simulink model "DeltaQuad"  (Simulink 9.1)
settings: Solver=VariableStepAuto  StartTime=0.0  StopTime=10.0  RelTol=1e-3
settings Model: Creator=PSere  LastModifiedBy=PSere
settings DataIOCC: SaveFormat=Dataset
settings OptimizationCC: LifeSpan=auto
settings DebuggingCC: UnderspecifiedInitializationDetection=Simplified  MergeDetectMultiDrivingBlocksExec=error  SFUnexpectedBacktrackingDiag=error  SFNoUnconditionalDefaultTransitionDiag=error  SFExecutionAtInitializationDiag=warning
settings HardwareCC: ProdBitPerPointer=64  ProdBitPerSizeT=64  ProdBitPerPtrDiffT=64  ProdLargestAtomicFloat=Float  ProdIntDivRoundTo=Zero  ProdEndianess=LittleEndian  ProdWordSize=64  ProdHWDeviceType=Intel->x86-64 (Windows64)
settings ModelReferenceCC: PropagateSignalLabelsOutOfModel=on
settings CodeAppCC: StateflowObjectComments=off
settings GRTTargetCC: TargetLangStandard=C99 (ISO)  CombineOutputUpdateFcns=on  GRTInterface=off
settings ConfigComp: CovMetricSettings=dwe  CovHtmlReporting=off  CovSaveCumulativeToWorkspaceVar=off  CovSaveSingleToWorkspaceVar=off  CovExternalEMLEnable=on

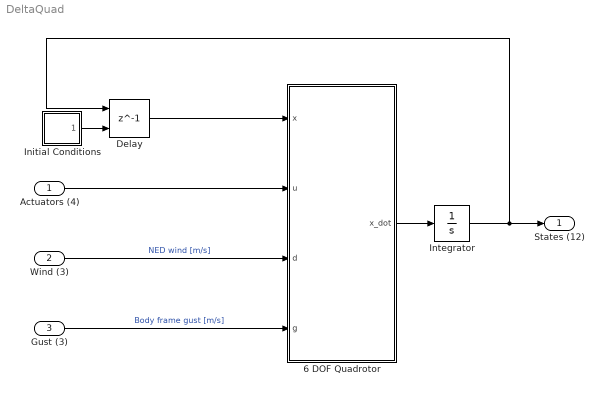
== system DeltaQuad ==
  Actuators (4) : Inport
  Wind (3) : Inport  Port=2
  Gust (3) : Inport  Port=3
  6 DOF Quadrotor : MATLAB Function  TreatAsAtomicUnit=on
  Delay : Delay  DelayLength=1  InitialConditionSource=Input port
      settings: InputPortMap=u0,p4
  "Initial Conditions " : Subsystem  mask{Pn=0, Pe=0, Pd=0, u=0, v=0, w=0, phi=0, theta=0, psi=0, p=0, q=0, r=0}
      mask prompts: Pn "Position North"; Pe "Position East"; Pd "Position Down"
  Integrator : Integrator
  States (12) : Outport
  wires:
  Actuators (4)/1 -> 6 DOF Quadrotor/2(u)
  Wind (3)/1 -> 6 DOF Quadrotor/3(d)  "NED wind [m/s]"
  Delay/1 -> 6 DOF Quadrotor/1(x)
  6 DOF Quadrotor/1(x_dot) -> Integrator/1
  Integrator/1 -> Delay/1, States (12)/1
  "Initial Conditions "/1(IC (12)) -> Delay/2
  Gust (3)/1 -> 6 DOF Quadrotor/4(g)  "Body frame gust [m/s]"

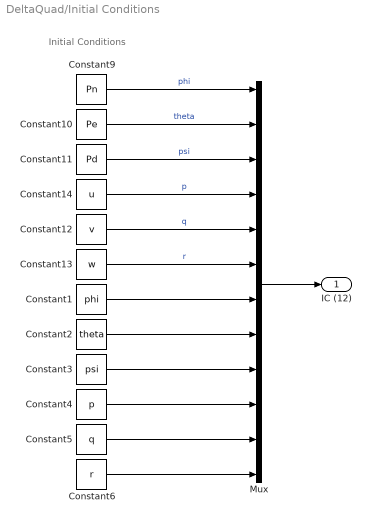
== system DeltaQuad/Initial Conditions  ==
  note: Initial Conditions
  Constant1 : Constant  Value=phi
  Constant10 : Constant  Value=Pe
  Constant11 : Constant  Value=Pd
  Constant12 : Constant  Value=v
  Constant13 : Constant  Value=w
  Constant14 : Constant  Value=u
  Constant2 : Constant  Value=theta
  Constant3 : Constant  Value=psi
  Constant4 : Constant  Value=p
  Constant5 : Constant  Value=q
  Constant6 : Constant  Value=r
  Constant9 : Constant  Value=Pn
  Mux : Mux  Inputs=12
  IC (12) : Outport
  wires:
  Constant14/1 -> Mux/4  "p"
  Constant12/1 -> Mux/5  "q"
  Constant11/1 -> Mux/3  "psi"
  Constant9/1 -> Mux/1  "phi"
  Constant13/1 -> Mux/6  "r"
  Constant10/1 -> Mux/2  "theta"
  Mux/1 -> IC (12)/1
  Constant1/1 -> Mux/7
  Constant2/1 -> Mux/8
  Constant3/1 -> Mux/9
  Constant4/1 -> Mux/10
  Constant5/1 -> Mux/11
  Constant6/1 -> Mux/12

== matlab function 6 DOF Quadrotor ==
  data: x input double; u input double; x_dot output double; d input double; g input double
function x_dot  = f(x, u, d, g)
%% Deltaquad Parameters:
I       = [ 0.115,  0,     -0.0015;
            0,      0.0576, 0;
           -0.0015, 0,      0.1712];       % moi matrix
       
Irzz    = 0.05;                            % rotor inertia
m       = 5.0;                             % mass
dx      = 0.35;                            % position of rotors x
dy      = 0.35;                            % position of rotors y
k1      = 12.2625;                         % N / kRPM^2
k2      = 4.2;                             % Nm / kRPM^2
S       = 0.5;                             % wing surface area
c       = 0.35;                            % MAC
b       = 0.2;                             % wing span

% Stability derivatives:
% Cl_0        =  -0.09167; % Zagi flying wing from "Beard small unmanned aircraft"
% Cl_beta     =  -0.0993;  % "Estimation of lateral aerodynamic coefficients for Skywalker X8"
% Cm_0        = -0.02338; % Zagi flying wing from "Beard small unmanned aircraft"
% Cm_alpha    = -0.5675;  % Zagi flying wing from "Beard small unmanned aircraft"
% Cn_0        = 0;
% Cn_beta     = 0.583;    % "Estimation of lateral aerodynamic coefficients for Skywalker X8"

% Lift, Drag and Sideforce coefficients
CL_0 = 0.1;
CL_alpha = 0.11;
CD_0 = 0.01;
CD_alpha = 0.01;
CY_0 = 0;
CY_beta = 0;

% Stability Derivatives
Cl_0        = 0; 
Cl_beta     = 0;  
Cm_0        = 0; 
Cm_alpha    = 0;
Cn_0        = 0;
Cn_beta     = 0;

%% Sines and cosines and rotational matrix pre-compute

s_phi   = sin(x(7));
c_phi   = cos(x(7));
s_th    = sin(x(8));
c_th    = cos(x(8));
t_th    = tan(x(8));
s_psi   = sin(x(9));
c_psi   = cos(x(9));

R_i2b   =  [1, 0, 0;         0, c_phi, s_phi;    0, -s_phi, c_phi]*...
           [c_th, 0, -s_th;  0, 1, 0;            s_th, 0, c_th]*...
           [c_psi, s_psi,    0; -s_psi, c_psi,   0; 0, 0, 1];
       
     

%% Inputs w, and aero disturbances d 
w       = [u(1); u(2); u(3); u(4)];                                                 % Rotor kilo RPMS:

%% FORCES

% 1) Fa: Aero forces
wb      = [x(4); x(5); x(6)] - (R_i2b * [d(1);d(2);d(3)] + [g(1);g(2);g(3)]);       % Airspeed in body frame
V       = sqrt(wb(1)^2 + wb(2)^2 + wb(3)^2);                                        % TAS
alpha   = atan(wb(3)/wb(1));
beta    = asin(wb(2)/V);
qS      = 0.5 * 1.225 * V^2 * S;

D = (CD_0  + CD_alpha  * alpha ) * qS;
Y = (CY_0  + CY_beta   * beta  ) * qS;
L = (CL_0  + CL_alpha  * alpha ) * qS;

Fa = [cos(alpha)    0   -sin(alpha);
      0             1   0;
      sin(alpha)    0   cos(alpha)]*[-D; -Y; -L];

% 2) Fr: Rotors
Fr = [0; 0; -k1*sum(w.^2)];

% 3) Fg: Gravity
g  = 9.81;
Fg = [ -m * g *s_th;
        m * g *c_th * s_phi;
        m * g *c_th * c_phi];

F = Fa + Fr + Fg;

%% MOMENTS (inertial effect of rotors ignored /G2/)

% 1) Ma: Aerodynamic Moments:
Ma = [(Cl_0 + Cl_beta  * beta ) * qS * b; 
      (Cm_0 + Cm_alpha * alpha) * qS * c; 
      (Cn_0 + Cn_beta  * beta ) * qS * b];
% 2) Mc: Conrol moments:
Mc = [-dy*k1, dy*k1,  dy*k1, -dy*k1;
       dx*k1, dx*k1, -dx*k1, -dx*k1;
       k2,    -k2,    k2,      -k2]*w.^2;
% 3) Mr: Gyroscopic effect:
Mr = [ Irzz*x(11), -Irzz*x(11),  Irzz*x(11), -Irzz*x(11);
      -Irzz*x(10),  Irzz*x(10), -Irzz*x(10),  Irzz*x(10);
            0,       0,       0,       0]*w;

%% Equations of motion:
x_dot = zeros(12, 1);

x_dot(1:3) = R_i2b'*[x(4);x(5);x(6)];

x_dot(4:6) = [x(12)*x(5) - x(11)*x(6);...
              x(10)*x(6) - x(12)*x(4);...
              x(11)*x(4) - x(10)*x(5)] + (1/m)*F; 
          
x_dot(7:9) = [1     s_phi*t_th          c_phi*t_th  ;...
              0     c_phi               -s_phi      ;...
              0     s_phi/c_th          c_phi/c_th]     *   [x(10);x(11);x(12)];
          
x_dot(10:12) = (I)\(Ma+Mc-Mr-cross([x(10);x(11);x(12)], I*[x(10);x(11);x(12)]));

end
